simulink library "csu_lan_landed_state_determination_lib"  (R2015b)
settings: Solver=ode45  StartTime=0.0  StopTime=10.0  RelTol=1e-3
values from neighbouring files (symbols this model uses):
  ini_landed_flag = boolean(0)    [csu_ini_initial_conditions_init.m]
undefined symbols (not defined in the file or in its folder): central_body_flattening, central_body_radius, central_body_rotation_rate, mpl_footpad_plane_to_origin, mpl_launchstand_height
libraries: simulink x5, util_frame_rotation_lib x3, util_quat_lib x3, util_common_lib x2, util_info_lib x1
settings Model: Creator=escrane  LastModifiedBy=Mark Agbayani
settings DataIOCC: SaveFormat=Array
settings DebuggingCC: UnderspecifiedInitializationDetection=Classic  MergeDetectMultiDrivingBlocksExec=none  SolverPrmCheckMsg=warning  StateNameClashWarn=warning
settings HardwareCC: ProdBitPerPointer=32  ProdLargestAtomicFloat=None  ProdIntDivRoundTo=Undefined  ProdEndianess=Unspecified  ProdWordSize=32  ProdHWDeviceType=32-bit Generic
settings GRTTargetCC: GeneratePreprocessorConditionals=Disable all
settings ConfigComp: CovModelRefEnable=Off  CovSFcnEnable=off

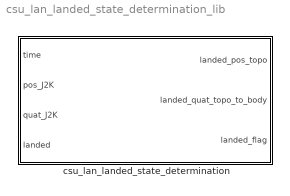
== system csu_lan_landed_state_determination_lib ==
  csu_lan_landed_state_determination : Subsystem

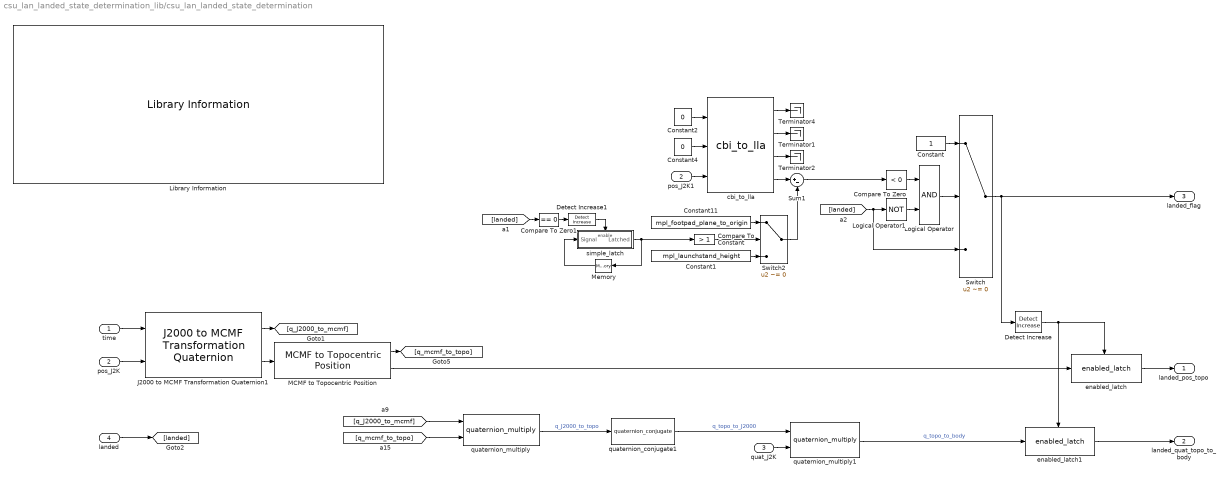
== system csu_lan_landed_state_determination_lib/csu_lan_landed_state_determination ==
  time : Inport
  pos_J2K : Inport  Port=2
  quat_J2K : Inport  Port=3
  landed : Inport  Port=4
  Compare To Constant : simulink/Logic and Bit Operations/Compare To Constant  relop=>  const=1  OutDataTypeStr=boolean
  Compare To Zero : simulink/Logic and Bit Operations/Compare To Zero  relop=<  OutDataTypeStr=boolean
  Compare To Zero1 : simulink/Logic and Bit Operations/Compare To Zero  relop===  OutDataTypeStr=boolean
  Constant : Constant  OutDataTypeStr=boolean
  Constant1 : Constant  Value=mpl_launchstand_height  VectorParams1D=off
  Constant11 : Constant  Value=mpl_footpad_plane_to_origin  VectorParams1D=off
  Constant2 : Constant  Value=0
  Constant4 : Constant  Value=0
  Detect Increase : simulink/Logic and Bit Operations/Detect Increase  vinit=ini_landed_flag  InputProcessing=Inherited  OutDataTypeStr=boolean
  Detect Increase1 : simulink/Logic and Bit Operations/Detect Increase  vinit=0  InputProcessing=Inherited  OutDataTypeStr=boolean
  J2000 to MCMF Transformation Quaternion1 : util_frame_rotation_lib/J2000 to MCMF  Transformation Quaternion  SystemSampleTime=-1
  Library Information : util_info_lib/Library Information  owner='escrane'
  Logical Operator : Logic  AllPortsSameDT=off  OutDataTypeStr=boolean
  Logical Operator1 : Logic  Operator=NOT  AllPortsSameDT=off  OutDataTypeStr=boolean
  MCMF to Topocentric Position : util_frame_rotation_lib/MCMF to Topocentric  Position  SystemSampleTime=-1
  Memory : Memory  InheritSampleTime=on
  Sum1 : Sum  Inputs=|+-
  Switch : Switch  Criteria=u2 ~= 0
  Switch2 : Switch  Criteria=u2 ~= 0
  Terminator1 : Terminator
  Terminator2 : Terminator
  Terminator4 : Terminator
  cbi_to_lla : util_frame_rotation_lib/cbi_to_lla  a=central_body_radius  b=central_body_radius*(1-central_body_flattening)  omega=central_body_rotation_rate(3)
  enabled_latch : util_common_lib/enabled_latch  initial_output=0
  enabled_latch1 : util_common_lib/enabled_latch  initial_output=0
  pos_J2K1 : InportShadow  Port=2
  quaternion_conjugate1 : util_quat_lib/quaternion_conjugate  SystemSampleTime=-1
  quaternion_multiply : util_quat_lib/quaternion_multiply  SystemSampleTime=-1
  quaternion_multiply1 : util_quat_lib/quaternion_multiply  SystemSampleTime=-1
  simple_latch : Subsystem
  landed_pos_topo : Outport
  landed_quat_topo_to_body : Outport  Port=2
  landed_flag : Outport  Port=3
  wires:
  cbi_to_lla/4 -> Sum1/1
  pos_J2K1/1 -> cbi_to_lla/3
  Constant2/1 -> cbi_to_lla/1
  cbi_to_lla/3 -> Terminator2/1
  cbi_to_lla/2 -> Terminator1/1
  cbi_to_lla/1 -> Terminator4/1
  Constant4/1 -> cbi_to_lla/2
  Constant1/1 -> Switch2/3
  Constant11/1 -> Switch2/1
  Switch2/1 -> Sum1/2
  Compare To Constant/1 -> Switch2/2
  Detect Increase1/1 -> simple_latch/Enable
  simple_latch/1(Latched) -> Memory/1, Compare To Constant/1
  Memory/1 -> simple_latch/1(Signal)
  Compare To Zero1/1 -> Detect Increase1/1
  [landed] -> Compare To Zero1/1
  landed/1 -> [landed]
  J2000 to MCMF Transformation Quaternion1/2 -> MCMF to Topocentric Position/1
  Detect Increase/1 -> enabled_latch/Enable, enabled_latch1/Enable
  Compare To Zero/1 -> Logical Operator/1
  MCMF to Topocentric Position/2 -> enabled_latch/1
  quat_J2K/1 -> quaternion_multiply1/2
  quaternion_conjugate1/1 -> quaternion_multiply1/1  "q_topo_to_J2000"
  quaternion_multiply/1 -> quaternion_conjugate1/1  "q_J2000_to_topo"
  [q_mcmf_to_topo] -> quaternion_multiply/2
  [q_J2000_to_mcmf] -> quaternion_multiply/1
  pos_J2K/1 -> J2000 to MCMF Transformation Quaternion1/2
  MCMF to Topocentric Position/1 -> [q_mcmf_to_topo]
  J2000 to MCMF Transformation Quaternion1/1 -> [q_J2000_to_mcmf]
  time/1 -> J2000 to MCMF Transformation Quaternion1/1
  [landed] -> Logical Operator1/1, Switch/3
  Logical Operator/1 -> Switch/2
  enabled_latch/1 -> landed_pos_topo/1
  quaternion_multiply1/1 -> enabled_latch1/1  "q_topo_to_body"
  enabled_latch1/1 -> landed_quat_topo_to_body/1
  Constant/1 -> Switch/1
  Logical Operator1/1 -> Logical Operator/2
  Switch/1 -> landed_flag/1, Detect Increase/1
  Sum1/1 -> Compare To Zero/1

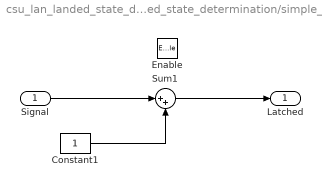
== system csu_lan_landed_state_determination_lib/csu_lan_landed_state_determination/simple_latch ==
  Signal : Inport
  Enable : EnablePort
  Constant1 : Constant
  Sum1 : Sum  Inputs=|++
  Latched : Outport  InitialOutput=0
  wires:
  Constant1/1 -> Sum1/2
  Sum1/1 -> Latched/1
  Signal/1 -> Sum1/1
